simulink model "EDDA_linear_IK"  (R2020a)
settings: Solver=ode45  StartTime=0.0  StopTime=T  FixedStep=0.4  RelTol=1e-6
values from neighbouring files (symbols this model uses):
  g = 9.81    [TestingIkRTR.m]    (also in TestingScript.m; TestingScriptRTR.m)
  Kd1 = Kp1/10    (= 100)    [TestingIkRTR.m]    (also in TestingScript.m; TestingScriptRTR.m)
  Kp1 = 1000    [TestingIkRTR.m]    (also in TestingScript.m; TestingScriptRTR.m)
  l2 = 0.3    [TestingIkRTR.m]    (also in TestingScriptRTR.m)
  O1 = 3.1    [TestingScript.m]
  O2 = 9.5    [TestingScript.m]
  O3 = 0.24    [TestingScript.m]
  O4 = 0.77    [TestingScript.m]
undefined symbols (not defined in the file or in its folder): gamma, l1
libraries: simulink x2
settings Model: Creator=ja  LastModifiedBy=ja

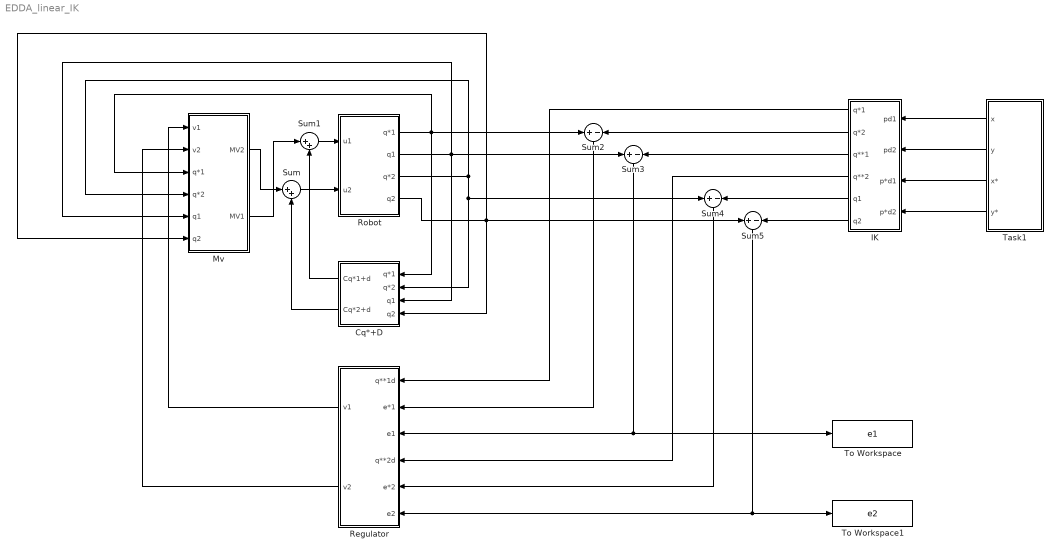
== system EDDA_linear_IK ==
  Cq*+D : Subsystem
  IK : Subsystem
  Mv : Subsystem
  Regulator : Subsystem
  Robot : Subsystem
  Sum : Sum  Inputs=|++
  Sum1 : Sum  Inputs=|++
  Sum{2..5} (4 alike) : Sum  Inputs=+-
  Task1 : Subsystem
  To Workspace : ToWorkspace  VariableName=e1  SampleTime=-1
  To Workspace1 : ToWorkspace  VariableName=e2  SampleTime=-1
  wires:
  Sum3/1 -> Regulator/3(e1), To Workspace/1
  Robot/3(q*2) -> Cq*+D/2(q*2), Sum4/1, Mv/4(q*2)
  Robot/4(q2) -> Cq*+D/4(q2), Mv/6(q2), Sum5/1
  IK/2(q*2) -> Sum2/2
  Sum5/1 -> To Workspace1/1, Regulator/6(e2)
  Robot/2(q1) -> Cq*+D/3(q1), Mv/5(q1), Sum3/1
  IK/3(q**1) -> Sum3/2
  IK/6(q2) -> Sum5/2
  Robot/1(q*1) -> Mv/3(q*1), Cq*+D/1(q*1), Sum2/1
  IK/5(q1) -> Sum4/2
  Sum1/1 -> Robot/1(u1)
  Sum/1 -> Robot/2(u2)
  Cq*+D/1(Cq*1+d) -> Sum1/2
  Cq*+D/2(Cq*2+d) -> Sum/2
  Regulator/2(v2) -> Mv/2(v2)
  Regulator/1(" v1") -> Mv/1(v1)
  Mv/1(MV2) -> Sum/1
  Mv/2(MV1) -> Sum1/1
  IK/1(q*1) -> Regulator/1(q**1d)
  Sum2/1 -> Regulator/2(e*1)
  IK/4(q**2) -> Regulator/4(q**2d)
  Sum4/1 -> Regulator/5(e*2)
  Task1/1(x) -> IK/1(pd1)
  Task1/4(y*) -> IK/4(p*d2)
  Task1/2(y) -> IK/2(pd2)
  Task1/3(x*) -> IK/3(p*d1)

== system EDDA_linear_IK/Cq*+D ==
  q*1 : Inport
  q*2 : Inport  Port=2
  q1 : Inport  Port=3
  q2 : Inport  Port=4
  C : Subsystem
  C1 : Subsystem
  D : Subsystem
  Sum2 : Sum  Inputs=+++
  Sum3 : Sum  Inputs=+++
  Cq*1+d : Outport
  Cq*2+d : Outport  Port=2
  wires:
  q2/1 -> C/4(q2), D/2(q2)
  D/1(Out1) -> Sum2/3
  q*1/1 -> C1/1(q*1), C/1(q*1)
  q1/1 -> C/2(q1), D/1(q1)
  q*2/1 -> C1/2(q*2), C/3(q*2)
  D/2(Out2) -> Sum3/3
  C/1(Out1) -> C1/3(C11)
  C/2(Out2) -> C1/4(C12)
  C/3(Out3) -> C1/5(C21)
  C/4(Out4) -> C1/6(C22)
  C1/4(Out4) -> Sum3/2
  C1/3(Out3) -> Sum3/1
  C1/1(Out1) -> Sum2/1
  C1/2(Out2) -> Sum2/2
  Sum3/1 -> Cq*2+d/1
  Sum2/1 -> Cq*1+d/1

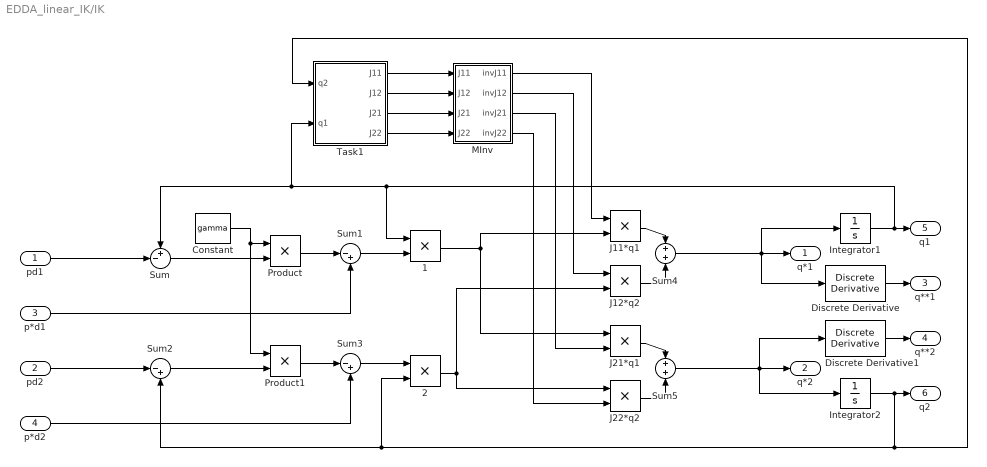
== system EDDA_linear_IK/IK ==
  pd1 : Inport
  pd2 : Inport  Port=2
  p*d1 : Inport  Port=3
  p*d2 : Inport  Port=4
  1 : Product
  2 : Product
  Constant : Constant  Value=gamma
  Discrete Derivative : simulink/Discrete/Discrete Derivative  gainval=1.0  ICPrevScaledInput=0.0  OutMin=[]  OutMax=[]  OutDataType=fixdt(1, 16)  OutScaling=2^-10  DoSatur=off
  Discrete Derivative1 : simulink/Discrete/Discrete Derivative  gainval=1.0  ICPrevScaledInput=0.0  OutMin=[]  OutMax=[]  OutDataType=fixdt(1, 16)  OutScaling=2^-10  DoSatur=off
  Integrator1 : Integrator  InitialCondition=0.1
  Integrator2 : Integrator  InitialCondition=0.1
  J11*q1 : Product
  J12*q2 : Product
  J21*q1 : Product
  J22*q2 : Product
  MInv : Subsystem
  Product : Product
  Product1 : Product
  Sum : Sum  Inputs=+-|
  Sum1 : Sum  Inputs=|-+
  Sum2 : Sum  Inputs=|-+
  Sum3 : Sum  Inputs=|-+
  Sum4 : Sum
  Sum5 : Sum
  Task1 : Subsystem
  q*1 : Outport
  q*2 : Outport  Port=2
  q**1 : Outport  Port=3
  q**2 : Outport  Port=4
  q1 : Outport  Port=5
  q2 : Outport  Port=6
  wires:
  Sum/1 -> Product/2
  Constant/1 -> Product1/1, Product/1
  pd1/1 -> Sum/2
  Product/1 -> Sum1/1
  p*d1/1 -> Sum1/2
  Product1/1 -> Sum3/1
  Sum2/1 -> Product1/2
  p*d2/1 -> Sum3/2
  Sum1/1 -> 1/2
  J12*q2/1 -> Sum4/2
  J11*q1/1 -> Sum4/1
  J22*q2/1 -> Sum5/2
  J21*q1/1 -> Sum5/1
  Sum4/1 -> Discrete Derivative/1, Integrator1/1, q*1/1
  Sum5/1 -> Discrete Derivative1/1, Integrator2/1, q*2/1
  2/1 -> J12*q2/2, J22*q2/1
  1/1 -> J21*q1/1, J11*q1/2
  MInv/1(invJ11) -> J11*q1/1
  MInv/2(invJ12) -> J12*q2/1
  MInv/3(invJ21) -> J21*q1/2
  MInv/4(invJ22) -> J22*q2/2
  Integrator1/1 -> q1/1, Task1/2(q1), Sum/1, 1/1
  pd2/1 -> Sum2/1
  Integrator2/1 -> q2/1, Sum2/2, 2/2, Task1/1(q2)
  Sum3/1 -> 2/1
  Discrete Derivative/1 -> q**1/1
  Discrete Derivative1/1 -> q**2/1
  Task1/1(J11) -> MInv/1(J11)
  Task1/3(J21) -> MInv/3(J21)
  Task1/2(J12) -> MInv/2(J12)
  Task1/4(J22) -> MInv/4(J22)

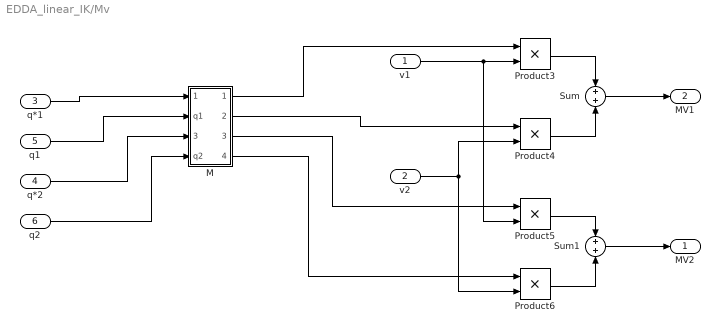
== system EDDA_linear_IK/Mv ==
  v1 : Inport
  v2 : Inport  Port=2
  q*1 : Inport  Port=3
  q*2 : Inport  Port=4
  q1 : Inport  Port=5
  q2 : Inport  Port=6
  M : Subsystem
  Product{3..6} (4 alike) : Product
  Sum : Sum
  Sum1 : Sum
  MV2 : Outport
  MV1 : Outport  Port=2
  wires:
  M/1(Out1) -> Product3/1
  Product6/1 -> Sum1/2
  Product3/1 -> Sum/1
  M/4(Out4) -> Product6/1
  Product4/1 -> Sum/2
  v2/1 -> Product4/2, Product6/2
  Product5/1 -> Sum1/1
  M/2(Out2) -> Product4/1
  v1/1 -> Product5/2, Product3/2
  M/3(Out3) -> Product5/1
  Sum/1 -> MV1/1
  Sum1/1 -> MV2/1
  q*1/1 -> M/1(q*1)
  q2/1 -> M/4(q2)
  q1/1 -> M/2(q1)
  q*2/1 -> M/3(q*2)

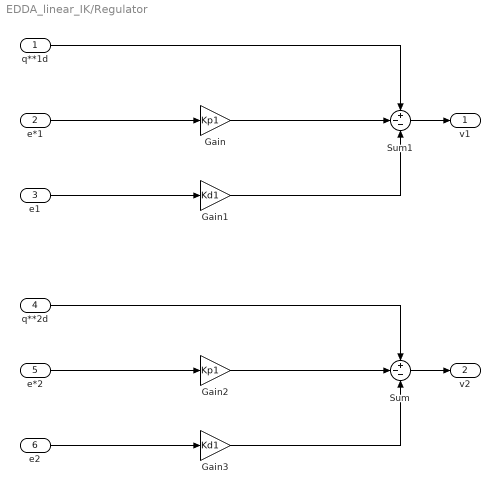
== system EDDA_linear_IK/Regulator ==
  q**1d : Inport
  e*1 : Inport  Port=2
  e1 : Inport  Port=3
  q**2d : Inport  Port=4
  e*2 : Inport  Port=5
  e2 : Inport  Port=6
  Gain : Gain  Gain=Kp1
  Gain1 : Gain  Gain=Kd1
  Gain2 : Gain  Gain=Kp1
  Gain3 : Gain  Gain=Kd1
  Sum : Sum  Inputs=+--
  Sum1 : Sum  Inputs=+--
  " v1" : Outport
  v2 : Outport  Port=2
  wires:
  Sum/1 -> v2/1
  Sum1/1 -> " v1"/1
  q**1d/1 -> Sum1/1
  q**2d/1 -> Sum/1
  e*1/1 -> Gain/1
  Gain/1 -> Sum1/2
  e1/1 -> Gain1/1
  Gain1/1 -> Sum1/3
  Gain2/1 -> Sum/2
  e*2/1 -> Gain2/1
  e2/1 -> Gain3/1
  Gain3/1 -> Sum/3

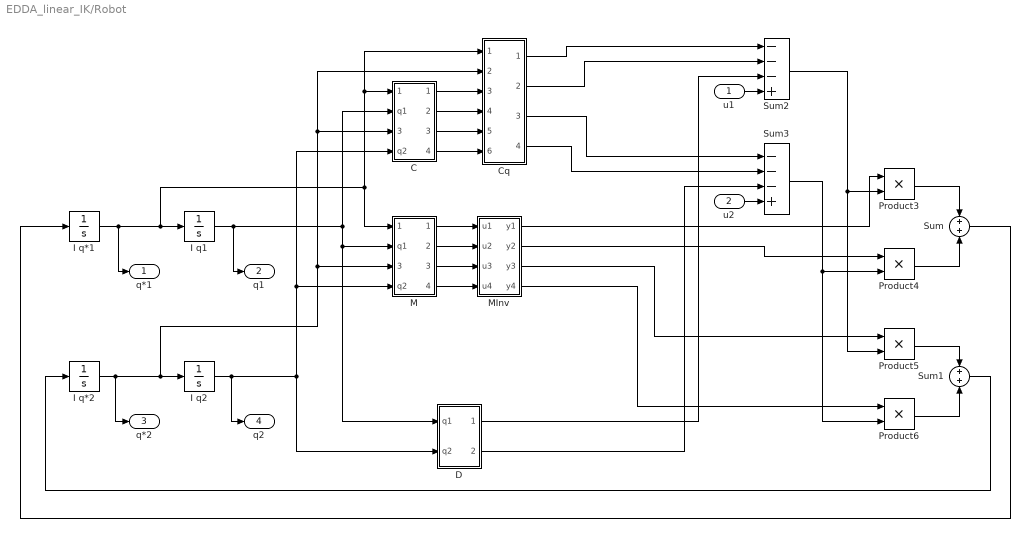
== system EDDA_linear_IK/Robot ==
  u1 : Inport
  u2 : Inport  Port=2
  C : Subsystem
  Cq : Subsystem
  D : Subsystem
  I q*1 : Integrator
  I q*2 : Integrator
  I q1 : Integrator
  I q2 : Integrator
  M : Subsystem
  MInv : Subsystem
  Product{3..6} (4 alike) : Product
  Sum : Sum
  Sum1 : Sum
  Sum2 : Sum  Inputs=---+
  Sum3 : Sum  Inputs=---+
  q*1 : Outport
  q1 : Outport  Port=2
  q*2 : Outport  Port=3
  q2 : Outport  Port=4
  wires:
  I q2/1 -> q2/1, C/4(q2), M/4(q2), D/2(q2)
  Sum/1 -> I q*1/1
  MInv/1(y1) -> Product3/1
  M/4(Out4) -> MInv/4(u4)
  D/1(Out1) -> Sum2/3
  I q*1/1 -> q*1/1, I q1/1, Cq/1(q*1), C/1(q*1), M/1(q*1)
  Sum1/1 -> I q*2/1
  I q1/1 -> q1/1, D/1(q1), M/2(q1), C/2(q1)
  Product6/1 -> Sum1/2
  Product3/1 -> Sum/1
  I q*2/1 -> q*2/1, M/3(q*2), Cq/2(q*2), C/3(q*2), I q2/1
  M/1(Out1) -> MInv/1(u1)
  MInv/4(y4) -> Product6/1
  Product4/1 -> Sum/2
  M/2(Out2) -> MInv/2(u2)
  D/2(Out2) -> Sum3/3
  Sum3/1 -> Product4/2, Product6/2
  Product5/1 -> Sum1/1
  u2/1 -> Sum3/4
  MInv/2(y2) -> Product4/1
  Sum2/1 -> Product5/2, Product3/2
  MInv/3(y3) -> Product5/1
  M/3(Out3) -> MInv/3(u3)
  u1/1 -> Sum2/4
  C/1(Out1) -> Cq/3(C11)
  C/2(Out2) -> Cq/4(C12)
  C/3(Out3) -> Cq/5(C21)
  C/4(Out4) -> Cq/6(C22)
  Cq/4(Out4) -> Sum3/2
  Cq/3(Out3) -> Sum3/1
  Cq/1(Out1) -> Sum2/1
  Cq/2(Out2) -> Sum2/2

== system EDDA_linear_IK/Task1 ==
  Clock : Clock
  Fcn1 : Fcn  Expr=-2*(pi^2)*cos(2*pi*u)
  Fcn3 : Fcn  Expr=-2*(pi^2)*sin(2*pi*u)
  Integrator1 : Integrator
  Integrator2 : Integrator  InitialCondition=1/4
  Integrator3 : Integrator  InitialCondition=2
  Integrator4 : Integrator
  To Workspace : ToWorkspace  VariableName=time  SaveFormat=Timeseries  SampleTime=-1
  x : Outport
  y : Outport  Port=2
  x* : Outport  Port=3
  y* : Outport  Port=4
  wires:
  Fcn1/1 -> Integrator2/1
  Clock/1 -> Fcn1/1, Fcn3/1, To Workspace/1
  Integrator2/1 -> Integrator4/1, x*/1
  Integrator1/1 -> Integrator3/1, y*/1
  Fcn3/1 -> Integrator1/1
  Integrator4/1 -> x/1
  Integrator3/1 -> y/1

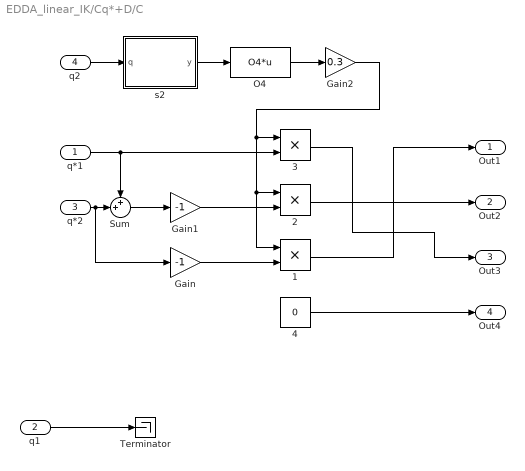
== system EDDA_linear_IK/Cq*+D/C ==
  q*1 : Inport
  q1 : Inport  Port=2
  q*2 : Inport  Port=3
  q2 : Inport  Port=4
  1 : Product
  2 : Product
  3 : Product
  4 : Constant  Value=0
  Gain : Gain  Gain=-1
  Gain1 : Gain  Gain=-1
  Gain2 : Gain  Gain=0.3
  O4 : Fcn  Expr=O4*u
  Sum : Sum  Inputs=++|
  Terminator : Terminator
  s2 : MATLAB Function  TreatAsAtomicUnit=on
  Out1 : Outport
  Out2 : Outport  Port=2
  Out3 : Outport  Port=3
  Out4 : Outport  Port=4
  wires:
  q*2/1 -> Gain/1, Sum/2
  q2/1 -> s2/1(q)
  q*1/1 -> 3/2, Sum/1
  s2/1(y) -> O4/1
  O4/1 -> Gain2/1
  Sum/1 -> Gain1/1
  Gain1/1 -> 2/2
  Gain/1 -> 1/2
  Gain2/1 -> 1/1, 2/1, 3/1
  4/1 -> Out4/1
  1/1 -> Out1/1
  3/1 -> Out3/1
  2/1 -> Out2/1
  q1/1 -> Terminator/1

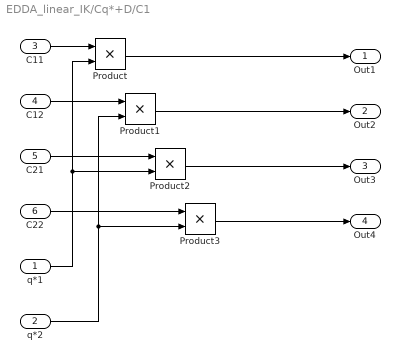
== system EDDA_linear_IK/Cq*+D/C1 ==
  q*1 : Inport
  q*2 : Inport  Port=2
  C11 : Inport  Port=3
  C12 : Inport  Port=4
  C21 : Inport  Port=5
  C22 : Inport  Port=6
  Product{,1..3} (4 alike) : Product
  Out1 : Outport
  Out2 : Outport  Port=2
  Out3 : Outport  Port=3
  Out4 : Outport  Port=4
  wires:
  C11/1 -> Product/1
  C12/1 -> Product1/1
  C21/1 -> Product2/1
  C22/1 -> Product3/1
  q*1/1 -> Product2/2, Product/2
  q*2/1 -> Product3/2, Product1/2
  Product3/1 -> Out4/1
  Product2/1 -> Out3/1
  Product1/1 -> Out2/1
  Product/1 -> Out1/1

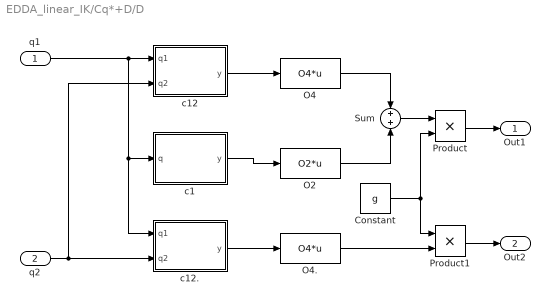
== system EDDA_linear_IK/Cq*+D/D ==
  q1 : Inport
  q2 : Inport  Port=2
  Constant : Constant  Value=g
  O2 : Fcn  Expr=O2*u
  O4 : Fcn  Expr=O4*u
  O4. : Fcn  Expr=O4*u
  Product : Product
  Product1 : Product
  Sum : Sum
  c1 : MATLAB Function  TreatAsAtomicUnit=on
  c12 : MATLAB Function  TreatAsAtomicUnit=on
  c12. : MATLAB Function  TreatAsAtomicUnit=on
  Out1 : Outport
  Out2 : Outport  Port=2
  wires:
  q1/1 -> c12./1(q1), c1/1(q), c12/1(q1)
  q2/1 -> c12./2(q2), c12/2(q2)
  c12./1(y) -> O4./1
  Product/1 -> Out1/1
  Sum/1 -> Product/1
  Product1/1 -> Out2/1
  Constant/1 -> Product/2, Product1/1
  O4./1 -> Product1/2
  c12/1(y) -> O4/1
  c1/1(y) -> O2/1
  O2/1 -> Sum/2
  O4/1 -> Sum/1

== system EDDA_linear_IK/IK/MInv ==
  J11 : Inport
  J12 : Inport  Port=2
  J21 : Inport  Port=3
  J22 : Inport  Port=4
  MInv : MATLAB Function  TreatAsAtomicUnit=on
  invJ11 : Outport
  invJ12 : Outport  Port=2
  invJ21 : Outport  Port=3
  invJ22 : Outport  Port=4
  wires:
  J22/1 -> MInv/4(u4)
  J21/1 -> MInv/3(u3)
  J12/1 -> MInv/2(u2)
  J11/1 -> MInv/1(u1)
  MInv/1(y1) -> invJ11/1
  MInv/2(y2) -> invJ12/1
  MInv/3(y3) -> invJ21/1
  MInv/4(y4) -> invJ22/1

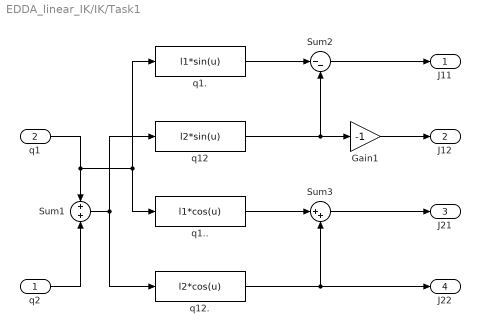
== system EDDA_linear_IK/IK/Task1 ==
  q2 : Inport
  q1 : Inport  Port=2
  Gain1 : Gain  Gain=-1
  Sum1 : Sum
  Sum2 : Sum  Inputs=|--
  Sum3 : Sum  Inputs=|++
  q1. : Fcn  Expr=l1*sin(u)
  q1.. : Fcn  Expr=l1*cos(u)
  q12 : Fcn  Expr=l2*sin(u)
  q12. : Fcn  Expr=l2*cos(u)
  J11 : Outport
  J12 : Outport  Port=2
  J21 : Outport  Port=3
  J22 : Outport  Port=4
  wires:
  q1/1 -> q1../1, q1./1, Sum1/1
  q2/1 -> Sum1/2
  q1./1 -> Sum2/1
  q12/1 -> Gain1/1, Sum2/2
  Sum2/1 -> J11/1
  Gain1/1 -> J12/1
  q1../1 -> Sum3/1
  q12./1 -> J22/1, Sum3/2
  Sum3/1 -> J21/1
  Sum1/1 -> q12/1, q12./1

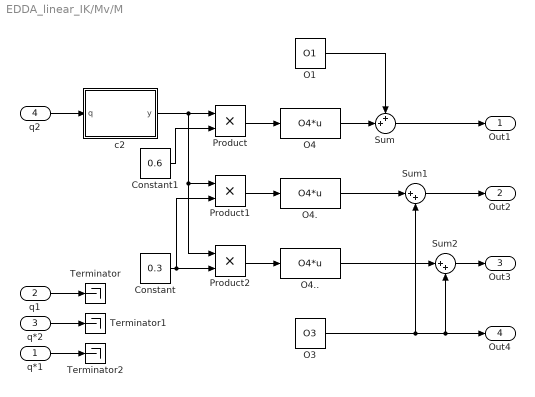
== system EDDA_linear_IK/Mv/M ==
  q*1 : Inport
  q1 : Inport  Port=2
  q*2 : Inport  Port=3
  q2 : Inport  Port=4
  Constant : Constant  Value=0.3
  Constant1 : Constant  Value=0.6
  O1 : Constant  Value=O1
  O3 : Constant  Value=O3
  O4 : Fcn  Expr=O4*u
  O4. : Fcn  Expr=O4*u
  O4.. : Fcn  Expr=O4*u
  Product : Product
  Product1 : Product
  Product2 : Product
  Sum : Sum  Inputs=++|
  Sum1 : Sum  Inputs=|++
  Sum2 : Sum  Inputs=|++
  Terminator : Terminator
  Terminator1 : Terminator
  Terminator2 : Terminator
  c2 : MATLAB Function  TreatAsAtomicUnit=on
  Out1 : Outport
  Out2 : Outport  Port=2
  Out3 : Outport  Port=3
  Out4 : Outport  Port=4
  wires:
  q2/1 -> c2/1(q)
  c2/1(y) -> Product2/1, Product1/1, Product/1
  Constant1/1 -> Product/2
  Constant/1 -> Product1/2, Product2/2
  q1/1 -> Terminator/1
  q*2/1 -> Terminator1/1
  q*1/1 -> Terminator2/1
  Product/1 -> O4/1
  Product2/1 -> O4../1
  Product1/1 -> O4./1
  O4/1 -> Sum/2
  Sum/1 -> Out1/1
  Sum1/1 -> Out2/1
  Sum2/1 -> Out3/1
  O3/1 -> Sum1/2, Sum2/2, Out4/1
  O1/1 -> Sum/1
  O4./1 -> Sum1/1
  O4../1 -> Sum2/1

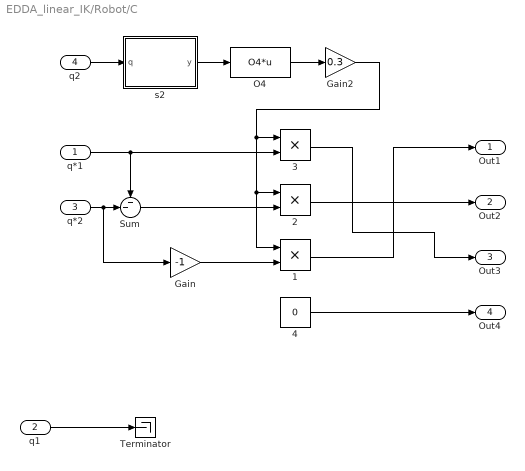
== system EDDA_linear_IK/Robot/C ==
  q*1 : Inport
  q1 : Inport  Port=2
  q*2 : Inport  Port=3
  q2 : Inport  Port=4
  1 : Product
  2 : Product
  3 : Product
  4 : Constant  Value=0
  Gain : Gain  Gain=-1
  Gain2 : Gain  Gain=0.3
  O4 : Fcn  Expr=O4*u
  Sum : Sum  Inputs=--|
  Terminator : Terminator
  s2 : MATLAB Function  TreatAsAtomicUnit=on
  Out1 : Outport
  Out2 : Outport  Port=2
  Out3 : Outport  Port=3
  Out4 : Outport  Port=4
  wires:
  q*2/1 -> Gain/1, Sum/2
  q2/1 -> s2/1(q)
  q*1/1 -> 3/2, Sum/1
  s2/1(y) -> O4/1
  O4/1 -> Gain2/1
  Sum/1 -> 2/2
  Gain/1 -> 1/2
  Gain2/1 -> 1/1, 2/1, 3/1
  4/1 -> Out4/1
  1/1 -> Out1/1
  3/1 -> Out3/1
  2/1 -> Out2/1
  q1/1 -> Terminator/1

== system EDDA_linear_IK/Robot/Cq ==
  q*1 : Inport
  q*2 : Inport  Port=2
  C11 : Inport  Port=3
  C12 : Inport  Port=4
  C21 : Inport  Port=5
  C22 : Inport  Port=6
  Product{,1..3} (4 alike) : Product
  Out1 : Outport
  Out2 : Outport  Port=2
  Out3 : Outport  Port=3
  Out4 : Outport  Port=4
  wires:
  C11/1 -> Product/1
  C12/1 -> Product1/1
  C21/1 -> Product2/1
  C22/1 -> Product3/1
  q*1/1 -> Product2/2, Product/2
  q*2/1 -> Product3/2, Product1/2
  Product3/1 -> Out4/1
  Product2/1 -> Out3/1
  Product1/1 -> Out2/1
  Product/1 -> Out1/1

== system EDDA_linear_IK/Robot/D ==
  q1 : Inport
  q2 : Inport  Port=2
  Constant : Constant  Value=g
  O2 : Fcn  Expr=O2*u
  O4 : Fcn  Expr=O4*u
  O4. : Fcn  Expr=O4*u
  Product : Product
  Product1 : Product
  Sum : Sum
  c1 : MATLAB Function  TreatAsAtomicUnit=on
  c12 : MATLAB Function  TreatAsAtomicUnit=on
  c12. : MATLAB Function  TreatAsAtomicUnit=on
  Out1 : Outport
  Out2 : Outport  Port=2
  wires:
  q1/1 -> c12./1(q1), c1/1(q), c12/1(q1)
  q2/1 -> c12./2(q2), c12/2(q2)
  c12./1(y) -> O4./1
  Product/1 -> Out1/1
  Sum/1 -> Product/1
  Product1/1 -> Out2/1
  Constant/1 -> Product/2, Product1/1
  O4./1 -> Product1/2
  c12/1(y) -> O4/1
  c1/1(y) -> O2/1
  O2/1 -> Sum/2
  O4/1 -> Sum/1

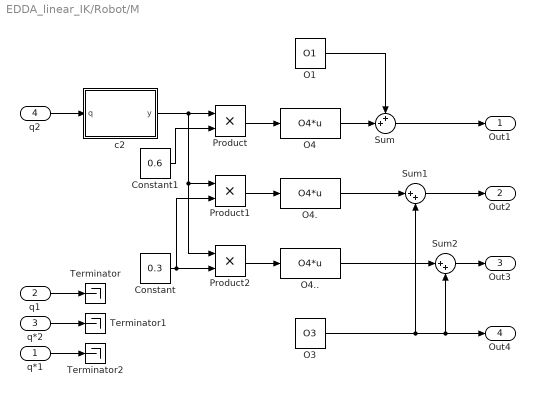
== system EDDA_linear_IK/Robot/M ==
  q*1 : Inport
  q1 : Inport  Port=2
  q*2 : Inport  Port=3
  q2 : Inport  Port=4
  Constant : Constant  Value=0.3
  Constant1 : Constant  Value=0.6
  O1 : Constant  Value=O1
  O3 : Constant  Value=O3
  O4 : Fcn  Expr=O4*u
  O4. : Fcn  Expr=O4*u
  O4.. : Fcn  Expr=O4*u
  Product : Product
  Product1 : Product
  Product2 : Product
  Sum : Sum  Inputs=++|
  Sum1 : Sum  Inputs=|++
  Sum2 : Sum  Inputs=|++
  Terminator : Terminator
  Terminator1 : Terminator
  Terminator2 : Terminator
  c2 : MATLAB Function  TreatAsAtomicUnit=on
  Out1 : Outport
  Out2 : Outport  Port=2
  Out3 : Outport  Port=3
  Out4 : Outport  Port=4
  wires:
  q2/1 -> c2/1(q)
  c2/1(y) -> Product2/1, Product1/1, Product/1
  Constant1/1 -> Product/2
  Constant/1 -> Product1/2, Product2/2
  q1/1 -> Terminator/1
  q*2/1 -> Terminator1/1
  q*1/1 -> Terminator2/1
  Product/1 -> O4/1
  Product2/1 -> O4../1
  Product1/1 -> O4./1
  O4/1 -> Sum/2
  Sum/1 -> Out1/1
  Sum1/1 -> Out2/1
  Sum2/1 -> Out3/1
  O3/1 -> Sum1/2, Sum2/2, Out4/1
  O1/1 -> Sum/1
  O4./1 -> Sum1/1
  O4../1 -> Sum2/1

== system EDDA_linear_IK/Robot/MInv ==
  u1 : Inport
  u2 : Inport  Port=2
  u3 : Inport  Port=3
  u4 : Inport  Port=4
  MInv : MATLAB Function  TreatAsAtomicUnit=on
  y1 : Outport
  y2 : Outport  Port=2
  y3 : Outport  Port=3
  y4 : Outport  Port=4
  wires:
  u4/1 -> MInv/4(u4)
  u3/1 -> MInv/3(u3)
  u2/1 -> MInv/2(u2)
  u1/1 -> MInv/1(u1)
  MInv/1(y1) -> y1/1
  MInv/2(y2) -> y2/1
  MInv/3(y3) -> y3/1
  MInv/4(y4) -> y4/1

== matlab function EDDA_linear_IK/Mv/M/c2 ==
  data: q input; y output
function y = c(q)

y = cos(q);

== matlab function EDDA_linear_IK/Robot/D/c12. ==
  data: q1 input; y output; q2 input
function y = c12(q1, q2)

y = cos(q1+q2);

== matlab function EDDA_linear_IK/Robot/D/c12 ==
  data: q1 input; y output; q2 input
function y = c12(q1, q2)

y = cos(q1+q2);

== matlab function EDDA_linear_IK/Robot/D/c1 ==
  data: q input; y output
function y = c(q)

y = cos(q);

== matlab function EDDA_linear_IK/Robot/M/c2 ==
  data: q input; y output
function y = c(q)

y = cos(q);

== matlab function EDDA_linear_IK/Robot/C/s2 ==
  data: q input; y output
function y = s(q)

y = sin(q);

== matlab function EDDA_linear_IK/Robot/MInv/MInv ==
  data: u1 input; y1 output; u2 input; u3 input; u4 input; y2 output; y3 output; y4 output
function [y1, y2, y3, y4] = c(u1, u2, u3, u4)

y = [u1 u2; u3 u4];
y = inv(y);

y1 = y(1);
y2 = y(2);
y3 = y(3);
y4 = y(4);

== matlab function EDDA_linear_IK/Cq*+D/C/s2 ==
  data: q input; y output
function y = s(q)

y = sin(q);

== matlab function EDDA_linear_IK/Cq*+D/D/c1 ==
  data: q input; y output
function y = c(q)

y = cos(q);

== matlab function EDDA_linear_IK/Cq*+D/D/c12 ==
  data: q1 input; y output; q2 input
function y = c12(q1, q2)

y = cos(q1+q2);

== matlab function EDDA_linear_IK/Cq*+D/D/c12. ==
  data: q1 input; y output; q2 input
function y = c12(q1, q2)

y = cos(q1+q2);

== matlab function EDDA_linear_IK/IK/MInv/MInv ==
  data: u1 input; y1 output; u2 input; u3 input; u4 input; y2 output; y3 output; y4 output
function [y1, y2, y3, y4] = c(u1, u2, u3, u4)

y = [u1 u2; u3 u4];
y = inv(y);

y1 = y(1);
y2 = y(2);
y3 = y(3);
y4 = y(4);
